simulink model "THREE_PH_PWM_INVERTER"  (R2023b)
settings: Solver=VariableStepAuto  StartTime=0.0  StopTime=0.5  RelTol=1e-3
libraries: spsIGBTDiodeLib x6, spsSeriesRLCBranchLib x3, simulink x3, spsVoltageMeasurementLib x3, spsDCVoltageSourceLib x1, sps_lib x1
settings Model: Creator=Ganga Srinivas  LastModifiedBy=Anusha

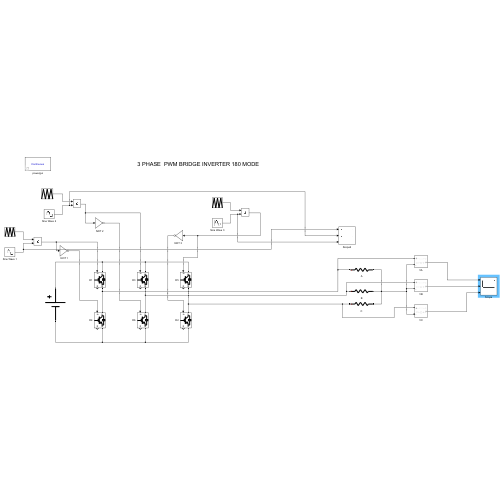
[thumbnail: Simulink's stored preview of the top-level diagram]
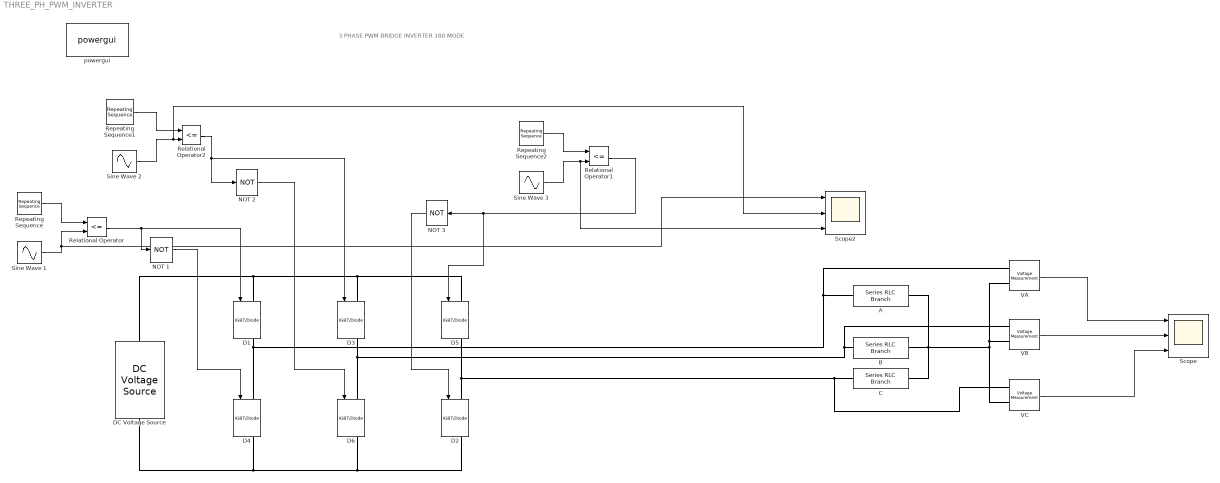
== system THREE_PH_PWM_INVERTER ==
  note: 3 PHASE PWM BRIDGE INVERTER 180 MODE
  A : spsSeriesRLCBranchLib/Series RLC Branch  LConnTagsString=__new0  RConnTagsString=__new0  BranchType=R  Resistance=100  Inductance=1e-3  SetiL0=off  InitialCurrent=0  Capacitance=1e-6  Setx0=off  InitialVoltage=0  Measurements=Branch voltage
  B : spsSeriesRLCBranchLib/Series RLC Branch  LConnTagsString=__new0  RConnTagsString=__new0  BranchType=R  Resistance=100  Inductance=1e-3  SetiL0=off  InitialCurrent=0  Capacitance=1e-6  Setx0=off  InitialVoltage=0  Measurements=Branch voltage
  C : spsSeriesRLCBranchLib/Series RLC Branch  LConnTagsString=__new0  RConnTagsString=__new0  BranchType=R  Resistance=100  Inductance=1e-3  SetiL0=off  InitialCurrent=0  Capacitance=1e-6  Setx0=off  InitialVoltage=0  Measurements=Branch voltage
  D{1..6} (6 alike) : spsIGBTDiodeLib/IGBT//Diode  Ron=1e-3  Rs=1e5  Cs=inf  Measurements=on
  DC Voltage Source : spsDCVoltageSourceLib/DC Voltage Source  Amplitude=100  Measurements=None
  NOT 1 : Logic  Operator=NOT  IconShape=distinctive  AllPortsSameDT=off  OutDataTypeStr=boolean
  NOT 2 : Logic  Operator=NOT  IconShape=distinctive  AllPortsSameDT=off  OutDataTypeStr=boolean
  NOT 3 : Logic  Operator=NOT  IconShape=distinctive  AllPortsSameDT=off  OutDataTypeStr=boolean
  Relational Operator : RelationalOperator  Operator=<=  OutDataTypeStr=boolean  RndMeth=Simplest  InputSameDT=off
  Relational Operator1 : RelationalOperator  Operator=<=  OutDataTypeStr=boolean  RndMeth=Simplest  InputSameDT=off
  Relational Operator2 : RelationalOperator  Operator=<=  OutDataTypeStr=boolean  RndMeth=Simplest  InputSameDT=off
  Repeating Sequence : simulink/Sources/Repeating Sequence  rep_seq_t=[0 1 2]  rep_seq_y=[0 2 0]
  Repeating Sequence1 : simulink/Sources/Repeating Sequence  rep_seq_t=[0 1 2]  rep_seq_y=[0 2 0]
  Repeating Sequence2 : simulink/Sources/Repeating Sequence  rep_seq_t=[0 1 2]  rep_seq_y=[0 2 0]
  Scope : Scope  NumInputPorts=3
  Scope2 : Scope  NumInputPorts=3
  Sine Wave 1 : Sin  Frequency=314.159  SampleTime=1e-6
  Sine Wave 2 : Sin  Frequency=314.159  Phase=2.094  SampleTime=1e-6
  Sine Wave 3 : Sin  Frequency=314.159  Phase=4.188  SampleTime=1e-6
  VA : spsVoltageMeasurementLib/Voltage Measurement  PhasorSimulation=off  OutputType=Complex  PSBequivalent=0
  VB : spsVoltageMeasurementLib/Voltage Measurement  PhasorSimulation=off  OutputType=Complex  PSBequivalent=0
  VC : spsVoltageMeasurementLib/Voltage Measurement  PhasorSimulation=off  OutputType=Complex  PSBequivalent=0
  powergui : sps_lib/powergui  Priority=1  SimulationMode=Continuous  SampleTime=50e-6  frequency=60  Iterations=50  frequencyindice=0  Pbase=100e6  ErrMax=1e-4  UnitsV=kV  UnitsW=MW  buscounter=0  FunctionMessages=off  echomessages=off  EnableUseOfTLC=off  CurrentSourceSwitches=off  DisableSnubberDevices=off  DisableRonSwitches=off  DisableVfSwitches=off  DisplayEquations=off  AutomaticDiscreteSolvers=off  SolverType=Tustin/Backward Euler (TBE)  Interpol=off  ExternalGateDelay=off  methode=off  Ts=100  x0status=blocks  SPID=on  SwTol=0  HookPort=off  NonlinearTolerance=1e-4  nMaxIteration=100  ContinueOnMaxIteration=off  RestoreLinks=warning  ResistiveCurrentMeasurement=off  Frange=[0:2:500]  Ylog=off  Xlog=on  ShowGrid=off  save=off  variable=ZData  structure=0  ZoomFFT=off  StartTime=0.0  cycles=1  DisplayStyle=1  fundamental=60  FreqAxis=off  MaxFrequency=1000  frequencyindicesteady=1  RmsSteady=1  display=off
  wires:
  NOT 1/1 -> D4/1
  Relational Operator/1 -> NOT 1/1, D1/1
  NOT 2/1 -> D6/1
  Relational Operator2/1 -> D3/1, NOT 2/1
  NOT 3/1 -> D2/1
  Relational Operator1/1 -> D5/1, NOT 3/1
  VA/1 -> Scope/1
  VB/1 -> Scope/2
  VC/1 -> Scope/3
  Repeating Sequence/1 -> Relational Operator/1
  Sine Wave 1/1 -> Relational Operator/2, Scope2/1
  Repeating Sequence2/1 -> Relational Operator1/1
  Sine Wave 3/1 -> Scope2/3, Relational Operator1/2
  Repeating Sequence1/1 -> Relational Operator2/1
  Sine Wave 2/1 -> Scope2/2, Relational Operator2/2
  connections:
  D2/LConn1 -- D5/RConn1 -- C/LConn1 -- VC/LConn1
  DC Voltage Source/RConn1 -- D1/LConn1 -- D3/LConn1 -- D5/LConn1
  DC Voltage Source/LConn1 -- D4/RConn1 -- D6/RConn1 -- D2/RConn1
  VC/LConn2 -- VB/LConn2 -- VA/LConn2 -- C/RConn1 -- A/RConn1 -- B/RConn1
  D3/RConn1 -- B/LConn1 -- VB/LConn1 -- D6/LConn1
  D4/LConn1 -- VA/LConn1 -- A/LConn1 -- D1/RConn1
